simulink model "amk_sim_model"  (R2022b)
settings: Solver=FixedStepAuto  StartTime=0.0  StopTime=4  FixedStep=1e-6  MaxStep=1e-5  MinStep=1e-6  RelTol=1e-3
values from neighbouring files (symbols this model uses):
  a_fw = log(9)/trfw    [amk_sim.m]    (also in amk_sim_2.m)
  ac = log(9)/tr    [amk_sim.m]    (also in amk_sim_2.m)
  ar_max = 1500    [amk_sim_2.m]
  as = log(9)/trs    [amk_sim.m]    (also in amk_sim_2.m)
  ba = 2*k^2*(as*J - 0)/(np^2*psi)    [amk_sim.m]    (also in amk_sim_2.m = 2*k^2*(as*J - bm)/(np^2*psi))
  bm = 0.02    [amk_sim.m]    (also in amk_sim_2.m = 0.008)
  I_base = 85.7    [amk_sim.m]    (also in amk_sim_2.m)
  I_max = 85.7    [amk_sim.m]    (also in amk_sim_2.m)
  Icon = 33.5    [amk_sim.m]    (also in amk_sim_2.m)
  Imax_interval = 1.24    [amk_sim.m]    (also in amk_sim_2.m = 5)
  Ipeak = 85.7    [amk_sim.m]    (also in amk_sim_2.m = 87.5)
  J = 2.5*(2.74e-4)    (= 0.000685)    [amk_sim.m]    (also in amk_sim_2.m = 0.000528)
  k = 1    [amk_sim.m]    (also in amk_sim_2.m)
  ki_ar = 0.2    [amk_sim_2.m]
  ki_s = 2*k^2*as^2*J/(np^2*psi)    [amk_sim.m]    (also in amk_sim_2.m)
  kp_ar = 1e-5    (= 1e-05)    [amk_sim_2.m]
  kp_s = 2*k^2*as*J/(np^2*psi)    [amk_sim.m]    (also in amk_sim_2.m)
  Ld = Ldm    (= 0.0004)    [amk_sim.m]    (also in amk_sim_2.m = 0.00012)
  Lq = Lqm    (= 0.00052)    [amk_sim.m]    (also in amk_sim_2.m = 0.00024)
  max_temp = 140    [amk_sim.m]    (also in amk_sim_2.m)
  np = 5    [amk_sim.m]    (also in amk_sim_2.m)
  Peak_power = 45000    [amk_sim.m]    (also in amk_sim_2.m = 50000)
  Peak_regen = -15000    [amk_sim.m]    (also in amk_sim_2.m = -1500000)
  psi = 0.047    [amk_sim.m]    (also in amk_sim_2.m = 0.05077789)
  rpm_nom = 20000    [amk_sim.m]    (also in amk_sim_2.m = 12000)
  Rs = 202.5e-3    (= 0.2025)    [amk_sim.m]    (also in amk_sim_2.m)
  sample_time = 1e-4    (= 0.0001)    [amk_sim.m]    (also in amk_sim_2.m = 1e-06)
  temp_threshold = 100    [amk_sim.m]    (also in amk_sim_2.m)
  u_dc = 550    [amk_sim.m]    (also in amk_sim_2.m)
  u_nom = u_dc*k    (= 550)    [amk_sim.m]    (also in amk_sim_2.m)
undefined symbols (not defined in the file or in its folder): sigbuilder_block
libraries: simulink x3
(part 5 of 5)

== matlab function amk_sim_model/pm flux est1 ==
  data: ar input; Imax input; imax output; ar_max input; imax_in input
function imax= fcn(ar, Imax, ar_max, imax_in)

if(ar <= (ar_max - 100) || ar <= 1)
    imax = Imax;
elseif((ar < ar_max) && (ar > (ar_max - 100)))
        if(imax_in < Imax)
            imax = imax_in + 0.01;
        else
            imax = Imax;
        end
else
    if(imax_in >= 0)
        imax = imax_in - 0.01;
    else
        imax = 0;
    end
end

== matlab function amk_sim_model/Subsystem1/pm flux est ==
  data: ar input; imax output; imax_prev input
function imax= fcn(ar, imax_prev)
imax = imax_prev;
if(ar > 6000)
    imax = imax_prev - 10;
end
if(ar < 4000)
    imax = imax_prev + 0.01;
end

if(imax > 85.7)
    imax = 85.7;
end
if(imax < 0)
    imax = 0;
end

== matlab function amk_sim_model/Current Controller/Subsystem/MATLAB Function1 ==
  data: vdc input; vdc_ramped output; vdc_ramped_previous input; vdc_actual input; sampling_time input; rise_time input; fall_time input
function vdc_ramped = fcn(vdc, vdc_ramped_previous, vdc_actual, sampling_time, rise_time, fall_time)

if(vdc_ramped_previous < (vdc + vdc_actual))
    vdc_ramped = vdc_ramped_previous + sampling_time*vdc_actual/rise_time;
else
    vdc_ramped = vdc_ramped_previous - sampling_time*vdc_actual/fall_time;
end

if(vdc_ramped > vdc_actual)
    vdc_ramped = vdc_actual;
end

== matlab function amk_sim_model/MATLAB Function ==
  data: n_max input; n_actual input; y output; y_prev input; Ts input; rise_time input
function y = fcn(n_max, n_actual, y_prev, Ts, rise_time)

if(y_prev < n_actual+300)
    y = y_prev + n_max*Ts/rise_time;
else
    y = n_actual+300;
end

if(y > 20000)
    y = 20000;
end
